simulink model "MMMS_v3"  (R2024b)
settings: Solver=VariableStepAuto  StartTime=0.0  StopTime=60  FixedStep=0.001  RelTol=1e-3
InitFcn:
  | %rho_0t=[0.29;0.29;0.29]; %m
  | %V_0t=[-0.001;-0.001;0];%[-0.0005;-0.0005;0];
  | %w_t=[0;0;-0.002];
  | 
  | 
  | %rho_0t=[0.3;0.3;0.2]; %m
  | %V_0t=[-0.001;-0.001;0];%[-0.0005;-0.0005;0];
  | %w_t=[0;0;-0.001];
values from neighbouring files (symbols this model uses):
  Dt = 0.1    [main_EKF.m]
  Fake_Manip_grad = -0.2.*eye(7)    [Initiate_FQ.m]
  g_cm = zeros(4,4,n)    [Initiate_KUKA_inv.m]    (also in Main_MMMS.m; test_KUKA_elements.m)
  g_It00 = [eye(3) rho_It;0 0 0 1]    [main_EKF.m]
  iota0 = eye(6,6)    [Initiate_KUKA_inv.m]    (also in Main_MMMS.m; test_KUKA_elements.m)
  K_d = 10*[1.3*eye(3) zeros(3);zeros(3) 0.8*eye(3)]    [Initiate_FQ.m]    (also in Initiate_KUKA_inv.m = 5*[0.7*eye(3) zeros(3);zeros(3) 0.5*eye(3)]; MMMS_Initiate_FQ.m; Main_MMMS.m = 5*[0.7*eye(3) zeros(3);zeros(3) 0.5*eye(3)]; test_KUKA_elements.m = 50*[0.7*eye(3) zeros(3);zeros(3) 0.5*eye(3)])
  K_i = 5*[0.1*eye(3) zeros(3);zeros(3) 0.01*eye(3)]    [Initiate_FQ.m]    (also in Initiate_KUKA_inv.m = 5*[0.01*eye(3) zeros(3);zeros(3) 0.001*eye(3)]; MMMS_Initiate_FQ.m; Main_MMMS.m = 5*[0.01*eye(3) zeros(3);zeros(3) 0.001*eye(3)]; test_KUKA_elements.m = 50*[0.01*eye(3) zeros(3);zeros(3) 0.001*eye(3)])
  K_p = 100*[0.1 0 0 0 0 0;0 0.1 0 0 0 0; 0 0 0.1 0 0 0; 0 0 0 0.01 0 0 ... (first row only)    [Initiate_FQ.m]    (also in Initiate_KUKA_inv.m = 5*[0.1 0 0 0 0 0;0 0.1 0 0 0 0; 0 0 0.1 0 0 0; 0 0 0 0.01 0 ; MMMS_Initiate_FQ.m; Main_MMMS.m = 5*[0.1 0 0 0 0 0;0 0.1 0 0 0 0; 0 0 0.1 0 0 0; 0 0 0 0.01 0 ; test_KUKA_elements.m = 50*[0.1 0 0 0 0 0;0 0.1 0 0 0 0; 0 0 0.1 0 0 0; 0 0 0 0.01 0)
  K_w = 200*eye(7)    [Initiate_FQ.m]    (also in MMMS_Initiate_FQ.m)
  K_wd = 2*eye(7)    [Initiate_FQ.m]    (also in MMMS_Initiate_FQ.m)
  m = randn(s,total_time_steps,6)*chol(R)    [main_EKF.m]
  M0 = M_temp.M0.data(:,:,1)    [Initiate_FQ.m]    (also in MMMS_Initiate_FQ.m; test_KUKA_elements.m)
  m0 = robot.Bodies{1,n+1}.Mass    [Initiate_KUKA_inv.m]    (also in Main_MMMS.m; test_KUKA_elements.m)
  m0_frak = diag_M(1:6,1:6)    [Initiate_KUKA_inv.m]    (also in Main_MMMS.m; make_uncertain.m = diag_M_unc(1:6,1:6); test_KUKA_elements.m)
  M0m = M_temp.M0m.data(:,:,1)    [Initiate_FQ.m]    (also in MMMS_Initiate_FQ.m; test_KUKA_elements.m)
  m_diag = diag_M(7:end,7:end)    [Initiate_KUKA_inv.m]    (also in Main_MMMS.m; make_uncertain.m = diag_M_unc(7:end,7:end); test_KUKA_elements.m)
  M_t = (((Adjoint(g_It))'\M_t_body)/(Adjoint(g_It)))    [Initiate_FQ.m]    (also in Initiate_KUKA_inv.m = [eye(3)*mt zeros(3); zeros(3) eye(3)*80]; MMMS_Initiate_FQ.m; Main_MMMS.m = [eye(3)*mt zeros(3); zeros(3) eye(3)*80]; test_KUKA_elements.m = [eye(3)*mt zeros(3); zeros(3) eye(3)*80])
  M_t_body = [eye(3)*mt zeros(3); zeros(3) eye(3)*0.416667]    [Initiate_FQ.m]    (also in MMMS_Initiate_FQ.m)
  mm = zeros(1,n)    [Initiate_KUKA_inv.m]    (also in Main_MMMS.m; test_KUKA_elements.m)
  mu = P0    [Initiate_FQ.m]    (also in Initiate_KUKA_inv.m = zeros(6,1); MMMS_Initiate_FQ.m; Main_MMMS.m = zeros(6,1); make_uncertain.m = P0_unc)
  mu_t = inv((Adjoint(g_It))')*M_t_body*[V_It;w_t]    [Initiate_FQ.m]    (also in Initiate_KUKA_inv.m = M_t*[V_0t;w_t]; MMMS_Initiate_FQ.m; Main_MMMS.m = M_t*[V_0t;w_t]; make_uncertain.m = inv((Adjoint(g_It))')*M_t_body_unc*[V_It;w_t])
  noise_st = 0.000005    (= 5e-06)    [main_EKF.m]
  q_dot_m = [0;0;0;0;0;0;0]    [Initiate_FQ.m]    (also in Initiate_KUKA_inv.m; MMMS_Initiate_FQ.m; Main_MMMS.m; test_KUKA_elements.m = [0])
  q_m = [0.2;1.2;0.3;2.5;0.5;1.5;0.6]    [Initiate_FQ.m]    (also in Initiate_KUKA_inv.m = [0;0;0;0;0;0;0]; MMMS_Initiate_FQ.m = [0.2;0.2;0.3;0.5;0.5;0.5;0.6]; Main_MMMS.m = [0;0;0;0;0;0;0]; test_KUKA_elements.m = [0.2;1.2;0.3;1.8;0.5;1.3;0.6])
  rho_It = [0;0;1.7]    [Initiate_FQ.m]    (also in MMMS_Initiate_FQ.m)
  s = RandStream.create('mrg32k3a','NumStreams',1)    [main_EKF.m]
  sc_size = 1    [Initiate_KUKA_inv.m]    (also in Main_MMMS.m; test_KUKA_elements.m)
  V_It = [0.0005;0.0005;0]    [Initiate_FQ.m]    (also in MMMS_Initiate_FQ.m = [0.001;0.001;0])
  Xi_m_matrix = zeros(6*n,n)    [Initiate_KUKA_inv.m]    (also in Main_MMMS.m)
undefined symbols (not defined in the file or in its folder): g_cm0, I0, Im, Mm, X, Xi_m, Y, Z
libraries: nesl_utility x314, sm_lib x231, robotcorelib x30, simulink x12
(part 7 of 13)

== system MMMS_v3/MMS4/Spacecraft ==
  Base1 : sm_lib/Body Elements/Brick Solid  BrickDimensions=[sc_size,sc_size,sc_size]  BrickDimensionsUnits=m  ExportEntireGeometry=off  InertiaType=Custom  BasedOnType=Mass  Density=1000  DensityUnits=kg/m^3  Mass=0  MassUnits=kg  CenterOfMass=[0 0 0]  CenterOfMassUnits=m  MomentsOfInertia=[0 0 0]  MomentsOfInertiaUnits=kg*m^2  ProductsOfInertia=[0 0 0]  ProductsOfInertiaUnits=kg*m^2  GraphicType=FromGeometry  MarkerShape=Sphere  MarkerSize=10  GraphicVisPropType=SimpleVisualProperties  GraphicDiffuseColor=[0.8 0.8 0.8]  GraphicOpacity=1  GraphicSpecularColor=[0.5 0.5 0.5 1.0]  GraphicAmbientColor=[0.15 0.15 0.15 1.0]  GraphicEmissiveColor=[0.0 0.0 0.0 1.0]  GraphicShininess=75  DoExposeReferenceFrame=on  SerializedFrames=<Frames><Frame><Id>Frame1</Id><Value><Name>F1</Name><Origin><Source>GeometricFeature</Source><FeatureName>+z surface</FeatureName></Origin><PrimaryAxis><DefinedDirection>+X</DefinedDirection><Source>ReferenceFrame</Source><SourceDirection>+X</SourceDirection><FeatureName></FeatureName></PrimaryAxis><SecondaryAxis><DefinedDirection>+Z</DefinedDirection><Source>ReferenceFrame</Source><SourceDirection>+Z</SourceDirection><FeatureName></FeatureName></SecondaryAxis></Value></Frame></Frames>
  Base2 : sm_lib/Body Elements/Brick Solid  Commented=on  BrickDimensions=[sc_size,sc_size,sc_size]  BrickDimensionsUnits=m  ExportEntireGeometry=off  InertiaType=CalculateFromGeometry  BasedOnType=Mass  Density=1000  DensityUnits=kg/m^3  Mass=10  MassUnits=kg  CenterOfMass=[0 0 0]  CenterOfMassUnits=m  MomentsOfInertia=[0 0 0]  MomentsOfInertiaUnits=kg*m^2  ProductsOfInertia=[0 0 0]  ProductsOfInertiaUnits=kg*m^2  GraphicType=FromGeometry  MarkerShape=Sphere  MarkerSize=10  GraphicVisPropType=SimpleVisualProperties  GraphicDiffuseColor=[0.5 0.5 0.5]  GraphicOpacity=1.0  GraphicSpecularColor=[0.5 0.5 0.5 1.0]  GraphicAmbientColor=[0.15 0.15 0.15 1.0]  GraphicEmissiveColor=[0.0 0.0 0.0 1.0]  GraphicShininess=75  DoExposeReferenceFrame=on  SerializedFrames=<Frames><Frame><Id>Frame1</Id><Value><Name>F1</Name><Origin><Source>GeometricFeature</Source><FeatureName>+z surface</FeatureName></Origin><PrimaryAxis><DefinedDirection>+X</DefinedDirection><Source>ReferenceFrame</Source><SourceDirection>+X</SourceDirection><FeatureName></FeatureName></PrimaryAxis><SecondaryAxis><DefinedDirection>+Z</DefinedDirection><Source>ReferenceFrame</Source><SourceDirection>+Z</SourceDirection><FeatureName></FeatureName></SecondaryAxis></Value></Frame></Frames>
  Cylindrical Solid : sm_lib/Body Elements/Cylindrical Solid  CylinderRadius=0.09  CylinderRadiusUnits=m  CylinderLength=0.15  CylinderLengthUnits=m  ExportEntireGeometry=off  InertiaType=CalculateFromGeometry  BasedOnType=Density  Density=0  DensityUnits=kg/m^3  Mass=1  MassUnits=kg  CenterOfMass=[0 0 0]  CenterOfMassUnits=m  MomentsOfInertia=[1 1 1]  MomentsOfInertiaUnits=kg*m^2  ProductsOfInertia=[0 0 0]  ProductsOfInertiaUnits=kg*m^2  GraphicType=FromGeometry  MarkerShape=Sphere  MarkerSize=10  GraphicVisPropType=SimpleVisualProperties  GraphicDiffuseColor=[0.8 0.8 0.8]  GraphicOpacity=1.0  GraphicSpecularColor=[0.5 0.5 0.5 1.0]  GraphicAmbientColor=[0.15 0.15 0.15 1.0]  GraphicEmissiveColor=[0.0 0.0 0.0 1.0]  GraphicShininess=75  DoExposeReferenceFrame=on  SerializedFrames=<Frames><Frame><Id>Frame1</Id><Value><Name>F1</Name><Origin><Source>GeometricFeature</Source><FeatureName>top surface</FeatureName></Origin><PrimaryAxis><DefinedDirection>+Z</DefinedDirection><Source>ReferenceFrame</Source><SourceDirection>+Z</SourceDirection><FeatureName></FeatureName></PrimaryAxis><SecondaryAxis><DefinedDirection>+X</DefinedDirection><Source>ReferenceFrame</Source><SourceDirection>+X</SourceDirection><FeatureName></FeatureName></SecondaryAxis></Value></Frame></Frames>
  Inertia : sm_lib/Body Elements/Inertia  InertiaType=Custom  Mass=mm(7)  MassUnits=kg  CenterOfMass=[0, 0, 0]  CenterOfMassUnits=m  MomentsOfInertia=[Im(1,1,7) Im(2,2,7) Im(3,3,7)]  MomentsOfInertiaUnits=kg*m^2  ProductsOfInertia=[Im(3,2,7) Im(3,1,7) Im(2,1,7)]  ProductsOfInertiaUnits=kg*m^2  GraphicType=None  MarkerShape=Inertia  MarkerSize=20  GraphicVisPropType=SimpleVisualProperties  GraphicDiffuseColor=[0.5 0.5 0.5]  GraphicOpacity=1.0  GraphicSpecularColor=[0.5 0.5 0.5 1.0]  GraphicAmbientColor=[0.15 0.15 0.15 1.0]  GraphicEmissiveColor=[0.0 0.0 0.0 1.0]  GraphicShininess=75
  Planar Joint : sm_lib/Joints/Planar Joint  JointMode=Normal  CompositeWrenchDir=FollowerOnBase  CompositeWrenchFrame=BaseFrame  SenseConstraintForce=off  SenseConstraintTorque=off  SenseTotalForce=off  SenseTotalTorque=off  PxPositionTargetSpecify=on  PxPositionTargetPriority=High  PxPositionTargetValue=0.75  PxPositionTargetValueUnits=m  PxVelocityTargetSpecify=off  PxVelocityTargetPriority=High  PxVelocityTargetValue=0  PxVelocityTargetValueUnits=m/s  PxEquilibriumPosition=0  PxEquilibriumPositionUnits=m  PxSpringStiffness=0  PxSpringStiffnessUnits=N/m  PxDampingCoefficient=0  PxDampingCoefficientUnits=N/(m/s)  PxLowerLimitSpecify=off  PxLowerLimitBound=-1  PxLowerLimitBoundUnits=m  PxLowerLimitStiffness=1e6  PxLowerLimitStiffnessUnits=N/m  PxLowerLimitDamping=1e3  PxLowerLimitDampingUnits=N/(m/s)  PxLowerLimitTransitionRegionWidth=1e-4  PxLowerLimitTransitionRegionWidthUnits=m  PxUpperLimitSpecify=off  PxUpperLimitBound=1  PxUpperLimitBoundUnits=m  PxUpperLimitStiffness=1e6  PxUpperLimitStiffnessUnits=N/m  PxUpperLimitDamping=1e3  PxUpperLimitDampingUnits=N/(m/s)  PxUpperLimitTransitionRegionWidth=1e-4  PxUpperLimitTransitionRegionWidthUnits=m  PxTorqueActuationMode=NoTorque  PxMotionActuationMode=ComputedMotion  PxSensePosition=off  PxSenseVelocity=off  PxSenseAcceleration=off  PxSenseTorqueForce=off  PxSenseLowerLimitTorqueForce=off  PxSenseUpperLimitTorqueForce=off  PyPositionTargetSpecify=on  PyPositionTargetPriority=High  PyPositionTargetValue=0  PyPositionTargetValueUnits=m  PyVelocityTargetSpecify=off  PyVelocityTargetPriority=High  PyVelocityTargetValue=0  PyVelocityTargetValueUnits=m/s  PyEquilibriumPosition=0  PyEquilibriumPositionUnits=m  PySpringStiffness=0  PySpringStiffnessUnits=N/m  PyDampingCoefficient=0  PyDampingCoefficientUnits=N/(m/s)  PyLowerLimitSpecify=off  PyLowerLimitBound=-1  PyLowerLimitBoundUnits=m  PyLowerLimitStiffness=1e6  PyLowerLimitStiffnessUnits=N/m  PyLowerLimitDamping=1e3  PyLowerLimitDampingUnits=N/(m/s)  PyLowerLimitTransitionRegionWidth=1e-4  PyLowerLimitTransitionRegionWidthUnits=m  PyUpperLimitSpecify=off  PyUpperLimitBound=1  PyUpperLimitBoundUnits=m  PyUpperLimitStiffness=1e6  PyUpperLimitStiffnessUnits=N/m  PyUpperLimitDamping=1e3  PyUpperLimitDampingUnits=N/(m/s)  PyUpperLimitTransitionRegionWidth=1e-4  PyUpperLimitTransitionRegionWidthUnits=m  PyTorqueActuationMode=NoTorque  PyMotionActuationMode=ComputedMotion  PySensePosition=off  PySenseVelocity=off  PySenseAcceleration=off  PySenseTorqueForce=off  PySenseLowerLimitTorqueForce=off  PySenseUpperLimitTorqueForce=off  RzPositionTargetSpecify=off  RzPositionTargetPriority=High  RzPositionTargetValue=-1  RzPositionTargetValueUnits=deg  RzVelocityTargetSpecify=off  RzVelocityTargetPriority=High  RzVelocityTargetValue=0  RzVelocityTargetValueUnits=deg/s  RzEquilibriumPosition=0  RzEquilibriumPositionUnits=deg  RzSpringStiffness=0  RzSpringStiffnessUnits=N*m/deg  RzDampingCoefficient=0  RzDampingCoefficientUnits=N*m/(deg/s)  RzLowerLimitSpecify=off  RzLowerLimitBound=-90  RzLowerLimitBoundUnits=deg  RzLowerLimitStiffness=1e4  RzLowerLimitStiffnessUnits=N*m/deg  RzLowerLimitDamping=10  RzLowerLimitDampingUnits=N*m/(deg/s)  RzLowerLimitTransitionRegionWidth=0.1  RzLowerLimitTransitionRegionWidthUnits=deg  RzUpperLimitSpecify=off  RzUpperLimitBound=90  RzUpperLimitBoundUnits=deg  RzUpperLimitStiffness=1e4  RzUpperLimitStiffnessUnits=N*m/deg  RzUpperLimitDamping=10  RzUpperLimitDampingUnits=N*m/(deg/s)  RzUpperLimitTransitionRegionWidth=0.1  RzUpperLimitTransitionRegionWidthUnits=deg  RzTorqueActuationMode=NoTorque  RzMotionActuationMode=ComputedMotion  RzSensePosition=off  RzSenseVelocity=off  RzSenseAcceleration=off  RzSenseTorqueForce=off  RzSenseLowerLimitTorqueForce=off  RzSenseUpperLimitTorqueForce=off
  Visual : sm_lib/Body Elements/File Solid  Commented=on  ExtGeomFileName=iiwa_description/meshes/iiwa7/visual/link_1.stl  UnitType=Custom  ExtGeomFileUnits=m  StepReaderType=HEX  ExportConvexHullGeometry=off  InertiaType=Custom  BasedOnType=DensityFromFile  Density=1000  DensityUnits=kg/m^3  Mass=0  MassUnits=kg  CenterOfMass=[0, 0, 0]  CenterOfMassUnits=m  MomentsOfInertia=[0, 0, 0]  MomentsOfInertiaUnits=kg*m^2  ProductsOfInertia=[0, 0, 0]  ProductsOfInertiaUnits=kg*m^2  GraphicType=FromGeometry  MarkerShape=Sphere  MarkerSize=10  GraphicVisPropType=SimpleVisualProperties  GraphicDiffuseColor=[1, 0.423529411765, 0.0392156862745]  GraphicOpacity=1  GraphicSpecularColor=[0.5 0.5 0.5 1.0]  GraphicAmbientColor=[0.15 0.15 0.15 1.0]  GraphicEmissiveColor=[0.0 0.0 0.0 1.0]  GraphicShininess=75  DoExposeReferenceFrame=on  SerializedFrames=<Frames/>
  VisualOriginTransform : sm_lib/Frames and Transforms/Rigid Transform  RotationMethod=RotationSequence  FollAlignAxisA=+X  BaseAlignAxisA=+Y  FollAlignAxisB=+Y  BaseAlignAxisB=+Z  RotationStandardAxis=+Z  RotationAngle=0.0  RotationAngleUnits=deg  RotationArbitraryAxis=[0 0 1]  RotationSequenceAxes=BaseAxes  RotationSequence=XYZ  RotationSequenceAngles=[0, 0, 0]  RotationSequenceAnglesUnits=rad  RotationMatrix=[1 0 0; 0 1 0; 0 0 1]  Quaternion=[1 0 0 0]  TranslationMethod=Cartesian  TranslationCartesianOffset=[0, 0, -0.15]  TranslationCartesianOffsetUnits=m  TranslationStandardAxis=+Z  TranslationStandardOffset=0  TranslationStandardOffsetUnits=m  TranslationROffset=0  TranslationROffsetUnits=m  TranslationThetaOffset=0  TranslationThetaOffsetUnits=deg  TranslationZOffset=0  TranslationZOffsetUnits=m
  iiwa_joint_2_OriginTransform : sm_lib/Frames and Transforms/Rigid Transform  RotationMethod=RotationMatrix  FollAlignAxisA=+X  BaseAlignAxisA=+Y  FollAlignAxisB=+Y  BaseAlignAxisB=+Z  RotationStandardAxis=+Z  RotationAngle=0.0  RotationAngleUnits=deg  RotationArbitraryAxis=[0 0 1]  RotationSequenceAxes=BaseAxes  RotationSequence=XYZ  RotationSequenceAngles=[1.57079632679, 0, 3.14159265359]  RotationSequenceAnglesUnits=rad  RotationMatrix=g_cm(1:3,1:3,7)  Quaternion=[1 0 0 0]  TranslationMethod=Cartesian  TranslationCartesianOffset=g_cm(1:3,4,7)'  TranslationCartesianOffsetUnits=m  TranslationStandardAxis=+Z  TranslationStandardOffset=0  TranslationStandardOffsetUnits=m  TranslationROffset=0  TranslationROffsetUnits=m  TranslationThetaOffset=0  TranslationThetaOffsetUnits=deg  TranslationZOffset=0  TranslationZOffsetUnits=m
  iiwa_joint_2_OriginTransform1 : sm_lib/Frames and Transforms/Rigid Transform  RotationMethod=RotationMatrix  FollAlignAxisA=+X  BaseAlignAxisA=+Y  FollAlignAxisB=+Y  BaseAlignAxisB=+Z  RotationStandardAxis=+Z  RotationAngle=0.0  RotationAngleUnits=deg  RotationArbitraryAxis=[0 0 1]  RotationSequenceAxes=BaseAxes  RotationSequence=XYZ  RotationSequenceAngles=[1.57079632679, 0, 3.14159265359]  RotationSequenceAnglesUnits=rad  RotationMatrix=g_cm(1:3,1:3,7)  Quaternion=[1 0 0 0]  TranslationMethod=Cartesian  TranslationCartesianOffset=g_cm(1:3,4,7)'  TranslationCartesianOffsetUnits=m  TranslationStandardAxis=+Z  TranslationStandardOffset=0  TranslationStandardOffsetUnits=m  TranslationROffset=0  TranslationROffsetUnits=m  TranslationThetaOffset=0  TranslationThetaOffsetUnits=deg  TranslationZOffset=0  TranslationZOffsetUnits=m
  F : PMIOPort  Side=Left
  F1 : PMIOPort  Port=2  Side=Right
  F3 : PMIOPort  Port=3  Side=Left
  connections:
  F3/RConn1 -- Planar Joint/LConn1
  iiwa_joint_2_OriginTransform/LConn1 -- Cylindrical Solid/LConn1 -- F1/RConn1
  iiwa_joint_2_OriginTransform1/LConn1 -- Inertia/RConn1 -- iiwa_joint_2_OriginTransform/RConn1 -- VisualOriginTransform/LConn1 -- F/RConn1
  Base1/RConn1 -- VisualOriginTransform/RConn1
  Planar Joint/RConn1 -- iiwa_joint_2_OriginTransform1/RConn1

== system MMMS_v3/MMS4/join//link 1 ==
  iiwa_joint_1 : sm_lib/Joints/Revolute Joint  JointMode=Normal  CompositeWrenchDir=FollowerOnBase  CompositeWrenchFrame=BaseFrame  SenseConstraintForce=off  SenseConstraintTorque=off  SenseTotalForce=off  SenseTotalTorque=off  PositionTargetSpecify=on  PositionTargetPriority=High  PositionTargetValue=q_m(7)  PositionTargetValueUnits=rad  VelocityTargetSpecify=on  VelocityTargetPriority=High  VelocityTargetValue=q_dot_m(7)  VelocityTargetValueUnits=rad/s  EquilibriumPosition=0  EquilibriumPositionUnits=deg  SpringStiffness=0  SpringStiffnessUnits=N*m/deg  DampingCoefficient=0  DampingCoefficientUnits=kg*m^2/(rad*s)  LowerLimitSpecify=off  LowerLimitBound=-2.96705972839  LowerLimitBoundUnits=rad  LowerLimitStiffness=1e4  LowerLimitStiffnessUnits=N*m/deg  LowerLimitDamping=10  LowerLimitDampingUnits=N*m/(deg/s)  LowerLimitTransitionRegionWidth=0.1  LowerLimitTransitionRegionWidthUnits=deg  UpperLimitSpecify=off  UpperLimitBound=2.96705972839  UpperLimitBoundUnits=rad  UpperLimitStiffness=1e4  UpperLimitStiffnessUnits=N*m/deg  UpperLimitDamping=10  UpperLimitDampingUnits=N*m/(deg/s)  UpperLimitTransitionRegionWidth=0.1  UpperLimitTransitionRegionWidthUnits=deg  TorqueActuationMode=InputTorque  MotionActuationMode=ComputedMotion  SensePosition=on  SenseVelocity=on  SenseAcceleration=on  SenseTorqueForce=off  SenseLowerLimitTorqueForce=off  SenseUpperLimitTorqueForce=off
  iiwa_link_1 : Subsystem
  b : PMIOPort  Side=Left
  f1 : PMIOPort  Port=2  Side=Left
  F1 : PMIOPort  Port=3  Side=Right
  q1 : PMIOPort  Port=4  Side=Right
  qd1 : PMIOPort  Port=5  Side=Right
  qdd1 : PMIOPort  Port=6  Side=Right
  connections:
  F1/RConn1 -- iiwa_link_1/RConn1
  iiwa_joint_1/RConn4 -- qdd1/RConn1
  iiwa_joint_1/RConn3 -- qd1/RConn1
  f1/RConn1 -- iiwa_joint_1/LConn2
  iiwa_joint_1/RConn2 -- q1/RConn1
  iiwa_joint_1/RConn1 -- b/RConn1
  iiwa_link_1/LConn1 -- iiwa_joint_1/LConn1

== system MMMS_v3/MMS4/joint//link2 ==
  iiwa_joint_2 : sm_lib/Joints/Revolute Joint  JointMode=Normal  CompositeWrenchDir=FollowerOnBase  CompositeWrenchFrame=BaseFrame  SenseConstraintForce=off  SenseConstraintTorque=off  SenseTotalForce=off  SenseTotalTorque=off  PositionTargetSpecify=on  PositionTargetPriority=High  PositionTargetValue=q_m(6)  PositionTargetValueUnits=rad  VelocityTargetSpecify=on  VelocityTargetPriority=High  VelocityTargetValue=q_dot_m(6)  VelocityTargetValueUnits=rad/s  EquilibriumPosition=0  EquilibriumPositionUnits=deg  SpringStiffness=0  SpringStiffnessUnits=N*m/deg  DampingCoefficient=0  DampingCoefficientUnits=kg*m^2/(rad*s)  LowerLimitSpecify=off  LowerLimitBound=-2.09439510239  LowerLimitBoundUnits=rad  LowerLimitStiffness=1e4  LowerLimitStiffnessUnits=N*m/deg  LowerLimitDamping=10  LowerLimitDampingUnits=N*m/(deg/s)  LowerLimitTransitionRegionWidth=0.1  LowerLimitTransitionRegionWidthUnits=deg  UpperLimitSpecify=off  UpperLimitBound=2.09439510239  UpperLimitBoundUnits=rad  UpperLimitStiffness=1e4  UpperLimitStiffnessUnits=N*m/deg  UpperLimitDamping=10  UpperLimitDampingUnits=N*m/(deg/s)  UpperLimitTransitionRegionWidth=0.1  UpperLimitTransitionRegionWidthUnits=deg  TorqueActuationMode=InputTorque  MotionActuationMode=ComputedMotion  SensePosition=on  SenseVelocity=on  SenseAcceleration=on  SenseTorqueForce=off  SenseLowerLimitTorqueForce=off  SenseUpperLimitTorqueForce=off
  iiwa_link_2 : Subsystem
  b : PMIOPort  Side=Left
  F1 : PMIOPort  Port=2  Side=Right
  f2 : PMIOPort  Port=3  Side=Left
  q2 : PMIOPort  Port=4  Side=Right
  qd2 : PMIOPort  Port=5  Side=Right
  qdd2 : PMIOPort  Port=6  Side=Right
  connections:
  iiwa_joint_2/RConn2 -- q2/RConn1
  f2/RConn1 -- iiwa_joint_2/LConn2
  iiwa_joint_2/RConn1 -- b/RConn1
  iiwa_joint_2/RConn4 -- qdd2/RConn1
  F1/RConn1 -- iiwa_link_2/RConn1
  iiwa_link_2/LConn1 -- iiwa_joint_2/LConn1
  iiwa_joint_2/RConn3 -- qd2/RConn1

== system MMMS_v3/MMS4/joint//link3 ==
  iiwa_joint_3 : sm_lib/Joints/Revolute Joint  JointMode=Normal  CompositeWrenchDir=FollowerOnBase  CompositeWrenchFrame=BaseFrame  SenseConstraintForce=off  SenseConstraintTorque=off  SenseTotalForce=off  SenseTotalTorque=off  PositionTargetSpecify=on  PositionTargetPriority=High  PositionTargetValue=q_m(5)  PositionTargetValueUnits=rad  VelocityTargetSpecify=on  VelocityTargetPriority=High  VelocityTargetValue=q_dot_m(5)  VelocityTargetValueUnits=rad/s  EquilibriumPosition=0  EquilibriumPositionUnits=deg  SpringStiffness=0  SpringStiffnessUnits=N*m/deg  DampingCoefficient=0  DampingCoefficientUnits=kg*m^2/(rad*s)  LowerLimitSpecify=off  LowerLimitBound=-2.96705972839  LowerLimitBoundUnits=rad  LowerLimitStiffness=1e4  LowerLimitStiffnessUnits=N*m/deg  LowerLimitDamping=10  LowerLimitDampingUnits=N*m/(deg/s)  LowerLimitTransitionRegionWidth=0.1  LowerLimitTransitionRegionWidthUnits=deg  UpperLimitSpecify=off  UpperLimitBound=2.96705972839  UpperLimitBoundUnits=rad  UpperLimitStiffness=1e4  UpperLimitStiffnessUnits=N*m/deg  UpperLimitDamping=10  UpperLimitDampingUnits=N*m/(deg/s)  UpperLimitTransitionRegionWidth=0.1  UpperLimitTransitionRegionWidthUnits=deg  TorqueActuationMode=InputTorque  MotionActuationMode=ComputedMotion  SensePosition=on  SenseVelocity=on  SenseAcceleration=on  SenseTorqueForce=off  SenseLowerLimitTorqueForce=off  SenseUpperLimitTorqueForce=off
  iiwa_link_3 : Subsystem
  b : PMIOPort  Side=Left
  F1 : PMIOPort  Port=2  Side=Right
  f3 : PMIOPort  Port=3  Side=Left
  q3 : PMIOPort  Port=4  Side=Right
  qd3 : PMIOPort  Port=5  Side=Right
  qdd3 : PMIOPort  Port=6  Side=Right
  connections:
  iiwa_joint_3/RConn1 -- b/RConn1
  f3/RConn1 -- iiwa_joint_3/LConn2
  F1/RConn1 -- iiwa_link_3/RConn1
  iiwa_joint_3/RConn2 -- q3/RConn1
  iiwa_joint_3/RConn3 -- qd3/RConn1
  iiwa_joint_3/RConn4 -- qdd3/RConn1
  iiwa_link_3/LConn1 -- iiwa_joint_3/LConn1

== system MMMS_v3/MMS4/joint//link4 ==
  iiwa_joint_4 : sm_lib/Joints/Revolute Joint  JointMode=Normal  CompositeWrenchDir=FollowerOnBase  CompositeWrenchFrame=BaseFrame  SenseConstraintForce=off  SenseConstraintTorque=off  SenseTotalForce=off  SenseTotalTorque=off  PositionTargetSpecify=on  PositionTargetPriority=High  PositionTargetValue=q_m(4)  PositionTargetValueUnits=rad  VelocityTargetSpecify=on  VelocityTargetPriority=High  VelocityTargetValue=q_dot_m(4)  VelocityTargetValueUnits=rad/s  EquilibriumPosition=0  EquilibriumPositionUnits=deg  SpringStiffness=0  SpringStiffnessUnits=N*m/deg  DampingCoefficient=0  DampingCoefficientUnits=kg*m^2/(rad*s)  LowerLimitSpecify=off  LowerLimitBound=-2.09439510239  LowerLimitBoundUnits=rad  LowerLimitStiffness=1e4  LowerLimitStiffnessUnits=N*m/deg  LowerLimitDamping=10  LowerLimitDampingUnits=N*m/(deg/s)  LowerLimitTransitionRegionWidth=0.1  LowerLimitTransitionRegionWidthUnits=deg  UpperLimitSpecify=off  UpperLimitBound=2.09439510239  UpperLimitBoundUnits=rad  UpperLimitStiffness=1e4  UpperLimitStiffnessUnits=N*m/deg  UpperLimitDamping=10  UpperLimitDampingUnits=N*m/(deg/s)  UpperLimitTransitionRegionWidth=0.1  UpperLimitTransitionRegionWidthUnits=deg  TorqueActuationMode=InputTorque  MotionActuationMode=ComputedMotion  SensePosition=on  SenseVelocity=on  SenseAcceleration=on  SenseTorqueForce=off  SenseLowerLimitTorqueForce=off  SenseUpperLimitTorqueForce=off
  iiwa_link_4 : Subsystem
  b : PMIOPort  Side=Left
  F1 : PMIOPort  Port=2  Side=Right
  f4 : PMIOPort  Port=3  Side=Left
  q4 : PMIOPort  Port=4  Side=Right
  qd4 : PMIOPort  Port=5  Side=Right
  qdd4 : PMIOPort  Port=6  Side=Right
  connections:
  iiwa_joint_4/RConn4 -- qdd4/RConn1
  iiwa_joint_4/RConn1 -- b/RConn1
  iiwa_joint_4/RConn2 -- q4/RConn1
  F1/RConn1 -- iiwa_link_4/RConn1
  f4/RConn1 -- iiwa_joint_4/LConn2
  iiwa_joint_4/RConn3 -- qd4/RConn1
  iiwa_link_4/LConn1 -- iiwa_joint_4/LConn1

== system MMMS_v3/MMS4/joint//link5 ==
  iiwa_joint_5 : sm_lib/Joints/Revolute Joint  JointMode=Normal  CompositeWrenchDir=FollowerOnBase  CompositeWrenchFrame=BaseFrame  SenseConstraintForce=off  SenseConstraintTorque=off  SenseTotalForce=off  SenseTotalTorque=off  PositionTargetSpecify=on  PositionTargetPriority=High  PositionTargetValue=q_m(3)  PositionTargetValueUnits=rad  VelocityTargetSpecify=on  VelocityTargetPriority=High  VelocityTargetValue=q_dot_m(3)  VelocityTargetValueUnits=rad/s  EquilibriumPosition=0  EquilibriumPositionUnits=rad  SpringStiffness=0  SpringStiffnessUnits=N*m/rad  DampingCoefficient=0  DampingCoefficientUnits=kg*m^2/(rad*s)  LowerLimitSpecify=off  LowerLimitBound=-2.96705972839  LowerLimitBoundUnits=rad  LowerLimitStiffness=1e4  LowerLimitStiffnessUnits=N*m/deg  LowerLimitDamping=10  LowerLimitDampingUnits=N*m/(deg/s)  LowerLimitTransitionRegionWidth=0.1  LowerLimitTransitionRegionWidthUnits=deg  UpperLimitSpecify=off  UpperLimitBound=2.96705972839  UpperLimitBoundUnits=rad  UpperLimitStiffness=1e4  UpperLimitStiffnessUnits=N*m/deg  UpperLimitDamping=10  UpperLimitDampingUnits=N*m/(deg/s)  UpperLimitTransitionRegionWidth=0.1  UpperLimitTransitionRegionWidthUnits=deg  TorqueActuationMode=InputTorque  MotionActuationMode=ComputedMotion  SensePosition=on  SenseVelocity=on  SenseAcceleration=on  SenseTorqueForce=off  SenseLowerLimitTorqueForce=off  SenseUpperLimitTorqueForce=off
  iiwa_link_5 : Subsystem
  b : PMIOPort  Side=Left
  F1 : PMIOPort  Port=2  Side=Right
  f5 : PMIOPort  Port=3  Side=Left
  q5 : PMIOPort  Port=4  Side=Right
  qd5 : PMIOPort  Port=5  Side=Right
  qdd5 : PMIOPort  Port=6  Side=Right
  connections:
  F1/RConn1 -- iiwa_link_5/RConn1
  f5/RConn1 -- iiwa_joint_5/LConn2
  iiwa_joint_5/RConn3 -- qd5/RConn1
  iiwa_link_5/LConn1 -- iiwa_joint_5/LConn1
  iiwa_joint_5/RConn4 -- qdd5/RConn1
  iiwa_joint_5/RConn2 -- q5/RConn1
  iiwa_joint_5/RConn1 -- b/RConn1

== system MMMS_v3/MMS4/joint//link6 ==
  PS-Simulink Converter1 : nesl_utility/PS-Simulink Converter  PhysicalDomain=network_engine_domain  SubClassName=ps_output  LeftPortType=input  RightPortType=output  PseudoPeriodic=off  Frequencies=[]  VectorFormat=1-D array  Unit=inherit  AffineConversion=off
  Scope : Scope
  iiwa_joint_6 : sm_lib/Joints/Revolute Joint  JointMode=Normal  CompositeWrenchDir=FollowerOnBase  CompositeWrenchFrame=BaseFrame  SenseConstraintForce=off  SenseConstraintTorque=off  SenseTotalForce=off  SenseTotalTorque=off  PositionTargetSpecify=on  PositionTargetPriority=High  PositionTargetValue=q_m(2)  PositionTargetValueUnits=rad  VelocityTargetSpecify=on  VelocityTargetPriority=High  VelocityTargetValue=q_dot_m(2)  VelocityTargetValueUnits=rad/s  EquilibriumPosition=0  EquilibriumPositionUnits=rad  SpringStiffness=0  SpringStiffnessUnits=N*m/rad  DampingCoefficient=0  DampingCoefficientUnits=kg*m^2/(rad*s)  LowerLimitSpecify=off  LowerLimitBound=-2.09439510239  LowerLimitBoundUnits=rad  LowerLimitStiffness=1e4  LowerLimitStiffnessUnits=N*m/deg  LowerLimitDamping=10  LowerLimitDampingUnits=N*m/(deg/s)  LowerLimitTransitionRegionWidth=0.1  LowerLimitTransitionRegionWidthUnits=deg  UpperLimitSpecify=off  UpperLimitBound=2.09439510239  UpperLimitBoundUnits=rad  UpperLimitStiffness=1e4  UpperLimitStiffnessUnits=N*m/deg  UpperLimitDamping=10  UpperLimitDampingUnits=N*m/(deg/s)  UpperLimitTransitionRegionWidth=0.1  UpperLimitTransitionRegionWidthUnits=deg  TorqueActuationMode=InputTorque  MotionActuationMode=ComputedMotion  SensePosition=on  SenseVelocity=on  SenseAcceleration=on  SenseTorqueForce=on  SenseLowerLimitTorqueForce=off  SenseUpperLimitTorqueForce=off
  iiwa_link_6 : Subsystem
  b : PMIOPort  Side=Left
  f6 : PMIOPort  Port=2  Side=Left
  F1 : PMIOPort  Port=3  Side=Right
  q6 : PMIOPort  Port=4  Side=Right
  qd6 : PMIOPort  Port=5  Side=Right
  qdd6 : PMIOPort  Port=6  Side=Right
  wires:
  PS-Simulink Converter1/1 -> Scope/1  "q_dot_1 to 3"
  connections:
  iiwa_joint_6/RConn5 -- PS-Simulink Converter1/LConn1
  iiwa_joint_6/RConn2 -- q6/RConn1
  iiwa_joint_6/RConn3 -- qd6/RConn1
  iiwa_joint_6/RConn4 -- qdd6/RConn1
  f6/RConn1 -- iiwa_joint_6/LConn2
  F1/RConn1 -- iiwa_link_6/RConn1
  iiwa_joint_6/RConn1 -- b/RConn1
  iiwa_link_6/LConn1 -- iiwa_joint_6/LConn1

== system MMMS_v3/MMS4/joint//link7 ==
  PS-Simulink Converter1 : nesl_utility/PS-Simulink Converter  PhysicalDomain=network_engine_domain  SubClassName=ps_output  LeftPortType=input  RightPortType=output  PseudoPeriodic=off  Frequencies=[]  VectorFormat=1-D array  Unit=inherit  AffineConversion=off
  Scope : Scope
  iiwa_joint_7 : sm_lib/Joints/Revolute Joint  JointMode=Normal  CompositeWrenchDir=FollowerOnBase  CompositeWrenchFrame=BaseFrame  SenseConstraintForce=off  SenseConstraintTorque=off  SenseTotalForce=off  SenseTotalTorque=off  PositionTargetSpecify=on  PositionTargetPriority=High  PositionTargetValue=q_m(1)  PositionTargetValueUnits=rad  VelocityTargetSpecify=on  VelocityTargetPriority=High  VelocityTargetValue=q_dot_m(1)  VelocityTargetValueUnits=rad/s  EquilibriumPosition=0  EquilibriumPositionUnits=rad  SpringStiffness=0  SpringStiffnessUnits=N*m/rad  DampingCoefficient=0  DampingCoefficientUnits=kg*m^2/(rad*s)  LowerLimitSpecify=off  LowerLimitBound=-3.05432619099  LowerLimitBoundUnits=rad  LowerLimitStiffness=1e4  LowerLimitStiffnessUnits=N*m/deg  LowerLimitDamping=10  LowerLimitDampingUnits=N*m/(deg/s)  LowerLimitTransitionRegionWidth=0.1  LowerLimitTransitionRegionWidthUnits=deg  UpperLimitSpecify=off  UpperLimitBound=3.05432619099  UpperLimitBoundUnits=rad  UpperLimitStiffness=1e4  UpperLimitStiffnessUnits=N*m/deg  UpperLimitDamping=10  UpperLimitDampingUnits=N*m/(deg/s)  UpperLimitTransitionRegionWidth=0.1  UpperLimitTransitionRegionWidthUnits=deg  TorqueActuationMode=InputTorque  MotionActuationMode=ComputedMotion  SensePosition=on  SenseVelocity=on  SenseAcceleration=on  SenseTorqueForce=on  SenseLowerLimitTorqueForce=off  SenseUpperLimitTorqueForce=off
  iiwa_link_7 : Subsystem
  b : PMIOPort  Side=Left
  f7 : PMIOPort  Port=2  Side=Left
  F1 : PMIOPort  Port=3  Side=Right
  q7 : PMIOPort  Port=4  Side=Right
  qd7 : PMIOPort  Port=5  Side=Right
  qdd7 : PMIOPort  Port=6  Side=Right
  wires:
  PS-Simulink Converter1/1 -> Scope/1  "q_dot_1 to 3"
  connections:
  iiwa_joint_7/RConn5 -- PS-Simulink Converter1/LConn1
  iiwa_joint_7/RConn1 -- b/RConn1
  F1/RConn1 -- iiwa_link_7/RConn1
  f7/RConn1 -- iiwa_joint_7/LConn2
  iiwa_joint_7/RConn3 -- qd7/RConn1
  iiwa_joint_7/RConn2 -- q7/RConn1
  iiwa_joint_7/RConn4 -- qdd7/RConn1
  iiwa_link_7/LConn1 -- iiwa_joint_7/LConn1

== system MMMS_v3/Controller23/Filter/Triggered Subsystem ==
  X_pos : Inport
  P_pos : Inport  Port=2
  Z : Inport  Port=3
  Trigger : TriggerPort  VariantControl=(inherit)  ShowOutputPort=on  SampleTimeType=periodic  SampleTime=0.5  InitialTriggerSignalState=positive
  Constant10 : Constant  Value=Dt
  Constant11 : Constant  Value=mu_t
  Constant12 : Constant  Value=noise_st.*eye(6)
  Constant13 : Constant  Value=noise_st.*eye(6)
  MATLAB Function : MATLAB Function  TreatAsAtomicUnit=on
  Mass : Constant  Value=[M_t(4:6,4:6) zeros(3); zeros(3) M_t(1:3,1:3)]
  Scope17 : Scope
  X_pos_out : Outport
  P_pos_out : Outport  Port=2
  wires:
  MATLAB Function/1(X_pos_out) -> X_pos_out/1
  Constant10/1 -> MATLAB Function/2(Dt)
  Mass/1 -> MATLAB Function/3(Mass_matrix)
  Constant13/1 -> MATLAB Function/8(R)
  Constant11/1 -> MATLAB Function/5(mu_vector)
  Constant12/1 -> MATLAB Function/7(Q)
  X_pos/1 -> MATLAB Function/4(X_pos)
  MATLAB Function/2(P_pos_out) -> P_pos_out/1
  P_pos/1 -> MATLAB Function/6(P_pos)
  Z/1 -> MATLAB Function/1(Z)
  Trigger/1 -> Scope17/1

== system MMMS_v3/Feedback Transformation/Inverse Dynamics1/C_hat ==
  note: C_hat
  q_m1 : Inport
  q_dot_m1 : Inport  Port=2
  A : Inport  Port=3
  <Lm0> : Inport  Port=4
  <Lm> : Inport  Port=5
  <M0> : Inport  Port=6
  <M0m> : Inport  Port=7
  <M0>1 : InportShadow  Port=6
  AMA_partial : MATLAB Function  TreatAsAtomicUnit=on
  A_partial : MATLAB Function  TreatAsAtomicUnit=on
  C_hat1 : MATLAB Function  TreatAsAtomicUnit=on
  Constant : Constant  Value=Xi_m
  Lm_partials : Subsystem
  M_partials : Subsystem
  Mm_hat_partial : MATLAB Function  TreatAsAtomicUnit=on
  M0_partial : Outport
  A_partial1 : Outport  Port=2
  C_hat : Outport  Port=3
  tag scope: A_partial=global, M0_partial=global
  wires:
  M_partials/3(Mm_partial) -> Mm_hat_partial/3(Mm_partial)
  Lm_partials/2(Lm0_partial) -> M_partials/3(Lm0_partial)
  q_m1/1 -> Lm_partials/1(q_m), Mm_hat_partial/1(q_m), C_hat1/1(q_m), AMA_partial/1(q_m), A_partial/1(q_m), M_partials/1(q_m)
  <M0m>/1 -> A_partial/5(M0m)
  Lm_partials/1(Lm_partial) -> M_partials/2(Lm_partial)
  M_partials/1(M0_partial) -> A_partial/3(M0_partial), M0_partial/1, AMA_partial/6(M0_partial), [M0_partial]
  A_partial/1(A_partial) -> AMA_partial/4(A_partial), [A_partial], A_partial1/1
  Constant/1 -> Lm_partials/2(Xi_m)
  M_partials/2(M0m_partial) -> A_partial/4(M0m_partial)
  Mm_hat_partial/1(Mm_hat_partial) -> C_hat1/2(Mm_hat_partial)
  q_dot_m1/1 -> C_hat1/3(q_dot_m)
  AMA_partial/1(AMA_partial) -> Mm_hat_partial/2(AMA_partial)
  <M0>/1 -> A_partial/2(M0)
  [V_I0] -> A_partial/6(V)
  [V_I0] -> M_partials/6(V)
  <Lm>/1 -> M_partials/4(Lm)
  [V_I0] -> AMA_partial/5(V)
  A/1 -> AMA_partial/3(A)
  C_hat1/1(C_hat) -> C_hat/1
  <M0>1/1 -> AMA_partial/2(M0)
  <Lm0>/1 -> M_partials/5(Lm0)

== system MMMS_v3/Feedback Transformation/Inverse Dynamics1/C_hat1 ==
  q_m : Inport
  q_dot_m : Inport  Port=2
  AMA_partial : MATLAB Function  TreatAsAtomicUnit=on
  A_partial : MATLAB Function  TreatAsAtomicUnit=on
  A_partial_par : MATLAB Function  TreatAsAtomicUnit=on
  Bus Selector : BusSelector  OutputSignals=M0,M0m
  Bus Selector1 : BusSelector  OutputSignals=Lm,Lm0
  C_hat : MATLAB Function  TreatAsAtomicUnit=on
  Constant : Constant  Value=Xi_m
  Constant2 : Constant  Commented=on  Value=m_diag  VectorParams1D=off
  Lm_partials : Subsystem
  M_partials : Subsystem
  Mm_hat_partial : MATLAB Function  TreatAsAtomicUnit=on
  M0_partial : Outport
  Out1 : Outport  Port=2
  C_hat1 : Outport  Port=3
  tag scope: A_partial=global, A_partial_par=global, M0_partial=global, Mm_partial=global
  wires:
  Bus Selector1/1 -> M_partials/4(Lm)  "<Lm>"
  M_partials/5(M0_partial_par) -> A_partial_par/7(M0_partial_par)
  M_partials/4(M0m_partial_par) -> A_partial_par/8(M0m_partial_par)
  M_partials/3(Mm_partial) -> [Mm_partial], Mm_hat_partial/3(Mm_partial)
  Lm_partials/4(Lm0_partial_par) -> M_partials/8(Lm0_partial_par)
  [L] -> Bus Selector1/1
  Bus Selector1/2 -> M_partials/5(Lm0)  "<Lm0>"
  AMA_partial/1(AMA_partial) -> Mm_hat_partial/2(AMA_partial)
  Lm_partials/2(Lm0_partial) -> M_partials/3(Lm0_partial)
  q_m/1 -> A_partial_par/1(q_m), AMA_partial/1(q_m), C_hat/1(q_m), Mm_hat_partial/1(q_m), A_partial/1(q_m), M_partials/1(q_m), Lm_partials/1(q_m)
  M_partials/1(M0_partial) -> AMA_partial/6(M0_partial), [M0_partial], M0_partial/1, A_partial/3(M0_partial), A_partial_par/3(M0_partial)
  Constant/1 -> Lm_partials/2(Xi_m)
  Mm_hat_partial/1(Mm_hat_partial) -> C_hat/2(Mm_hat_partial)
  Bus Selector/1 -> A_partial_par/2(M0), AMA_partial/2(M0), A_partial/2(M0)  "<M0>"
  [A_connection] -> AMA_partial/3(A)
  [V_Ie] -> AMA_partial/5(V)
  q_dot_m/1 -> C_hat/3(q_dot_m)
  [V_Ie] -> A_partial/6(V)
  [V_Ie] -> M_partials/7(V)
  Lm_partials/1(Lm_partial) -> M_partials/2(Lm_partial)
  Lm_partials/3(Lm_partial_par) -> M_partials/6(Lm_partial_par)
  [Mass_Matrix] -> Bus Selector/1
  [V_Ie] -> A_partial_par/6(V)
  Bus Selector/2 -> A_partial_par/5(M0m), A_partial/5(M0m)  "<M0m>"
  A_partial_par/1(A_partial_par) -> [A_partial_par]
  C_hat/1(C_hat) -> C_hat1/1
  M_partials/2(M0m_partial) -> A_partial_par/4(M0m_partial), A_partial/4(M0m_partial)
  A_partial/1(A_partial) -> Out1/1, [A_partial], AMA_partial/4(A_partial)

== system MMMS_v3/Feedback Transformation/Inverse Dynamics1/Inverse Dynamics ==
  note: Subsystem
  note: Inverse dynamics
  g_I0 : Inport
  <M0> : Inport  Port=2
  Mm : Inport  Port=3
  M0_dot : Inport  Port=4
  A_dot : Inport  Port=5
  C_hat : Inport  Port=6
  <M0>2 : InportShadow  Port=2
  Ad_g_I0_dot : MATLAB Function  TreatAsAtomicUnit=on
  Ad_g_I0_dot1 : MATLAB Function  TreatAsAtomicUnit=on
  Ad_g_te_dot : MATLAB Function  TreatAsAtomicUnit=on
  FU : MATLAB Function  TreatAsAtomicUnit=on
  Fm : MATLAB Function  TreatAsAtomicUnit=on
  Fmu : MATLAB Function  TreatAsAtomicUnit=on
  Gain : Gain  Commented=on  Gain=-1
  Goto : Goto  Commented=on  GotoTag=JJ  TagVisibility=global
  Inverse Dynamics : MATLAB Function  Commented=on  TreatAsAtomicUnit=on
  MATLAB Function3 : MATLAB Function  TreatAsAtomicUnit=on
  MmJcross : MATLAB Function  TreatAsAtomicUnit=on
  Mm_hat : MATLAB Function  TreatAsAtomicUnit=on
  Mt : Constant  Value=M_t
  Scope1 : Scope
  Scope2 : Scope
  F_U : Outport
  F_mu : Outport  Port=2
  F_t : Outport  Port=3
  F_m : Outport  Port=4
  tag scope: Mm_hat=global
  wires:
  Mm/1 -> Mm_hat/2(Mm)
  [A_connection] -> Mm_hat/3(A), MmJcross/2(A)
  FU/1(F_U) -> F_U/1
  Fmu/1(F_mu) -> F_mu/1
  MATLAB Function3/1(F_t) -> F_t/1
  Fm/1(F_m) -> F_m/1
  <M0>/1 -> Mm_hat/1(M0)
  C_hat/1 -> Fm/3(Cm_hat)
  <M0>2/1 -> Fmu/2(M0)
  g_I0/1 -> Fmu/4(g_I0), Ad_g_I0_dot/1(g_I0)
  M0_dot/1 -> Fmu/3(M_0_dot)
  A_dot/1 -> Fm/2(A_dot)
  [V_Ie] -> Ad_g_I0_dot/2(V_I0)
  Ad_g_I0_dot1/1(Ad_g_It_dot) -> MATLAB Function3/6(Ad_gIt_dot)
  Ad_g_I0_dot/1(Ad_g_I0_dot) -> Fmu/5(Ad_g_I0_dot)
  Ad_g_te_dot/1(Ad_g_te_dot) -> MATLAB Function3/5(Ad_gte_dot)
  [g_te] -> MATLAB Function3/2(g_te), Ad_g_te_dot/2(g_te)
  [g_It] -> MATLAB Function3/3(g_It), Ad_g_I0_dot1/2(g_It)
  [V_te] -> Ad_g_te_dot/1(V_te)
  [V_It] -> Ad_g_I0_dot1/1(V_t)
  Mt/1 -> MATLAB Function3/4(Mt)
  MmJcross/1(MmJcross) -> FU/1(MmJcross), MATLAB Function3/1(MmJcross), Fmu/1(MmJcross), Fm/1(MmJcross), Scope2/1
  Gain/1 -> Goto/1
  Mm_hat/1(Mm_hat) -> MmJcross/1(Mm_hat), [Mm_hat], Scope1/1

== system MMMS_v3/Feedback Transformation/Inverse Dynamics1/N_hat ==
  q_m : Inport
  q_dot_m : Inport  Port=2
  A : Inport  Port=3
  P : Inport  Port=4
  M0 : Inport  Port=5
  Constant : Constant  Value=iota0
  Matrix Multiply : Product  Multiplication=Matrix(*)
  N_hat : MATLAB Function  TreatAsAtomicUnit=on
  To Workspace : ToWorkspace  VariableName=N_firstpart  SaveFormat=Timeseries  SampleTime=-1
  N_hat1 : Outport
  wires:
  P/1 -> Matrix Multiply/2, N_hat/5(P)
  [M0_partial] -> N_hat/6(M0_partial)
  N_hat/1(N_hat_temp) -> To Workspace/1, Matrix Multiply/1
  q_m/1 -> N_hat/1(q_m)
  q_dot_m/1 -> N_hat/2(q_dot_m)
  [V_I0] -> N_hat/4(V)
  A/1 -> N_hat/3(A)
  [A_partial] -> N_hat/7(A_partial)
  Constant/1 -> N_hat/8(iota0)
  Matrix Multiply/1 -> N_hat1/1
  M0/1 -> N_hat/9(M0)

== system MMMS_v3/Feedback Transformation/Inverse Dynamics1/N_hat1 ==
  g_I0 : Inport
  q_m : Inport  Port=2
  q_dot_m : Inport  Port=3
  A : Inport  Port=4
  P : Inport  Port=5
  M0 : Inport  Port=6
  Constant : Constant  Value=iota0
  MATLAB Function : MATLAB Function  TreatAsAtomicUnit=on
  Matrix Multiply : Product  Multiplication=Matrix(*)
  N_hat : MATLAB Function  TreatAsAtomicUnit=on
  N_hat1 : Outport
  wires:
  [M0_partial] -> N_hat/6(M0_partial)
  N_hat/1(N_hat_temp) -> Matrix Multiply/1
  q_m/1 -> N_hat/1(q_m)
  q_dot_m/1 -> N_hat/2(q_dot_m)
  [V_Ie] -> MATLAB Function/2(V_Ie_e)
  A/1 -> N_hat/3(A)
  [A_partial] -> N_hat/7(A_partial)
  Constant/1 -> N_hat/8(iota0)
  Matrix Multiply/1 -> N_hat1/1
  M0/1 -> N_hat/9(M0)
  P/1 -> Matrix Multiply/2, N_hat/5(P)
  MATLAB Function/1(V_Ie) -> N_hat/4(V)
  g_I0/1 -> MATLAB Function/1(g_I0)

== system MMMS_v3/Feedback Transformation1/Inverse Dynamics1/C_hat ==
  note: C_hat
  q_m1 : Inport
  q_dot_m1 : Inport  Port=2
  A : Inport  Port=3
  <Lm0> : Inport  Port=4
  <Lm> : Inport  Port=5
  <M0> : Inport  Port=6
  <M0m> : Inport  Port=7
  <M0>1 : InportShadow  Port=6
  AMA_partial : MATLAB Function  TreatAsAtomicUnit=on
  A_partial : MATLAB Function  TreatAsAtomicUnit=on
  C_hat1 : MATLAB Function  TreatAsAtomicUnit=on
  Constant : Constant  Value=Xi_m
  Lm_partials : Subsystem
  M_partials : Subsystem
  Mm_hat_partial : MATLAB Function  TreatAsAtomicUnit=on
  M0_partial : Outport
  A_partial1 : Outport  Port=2
  C_hat : Outport  Port=3
  tag scope: A_partial=global, M0_partial=global
  wires:
  <Lm0>/1 -> M_partials/5(Lm0)
  <M0>1/1 -> AMA_partial/2(M0)
  C_hat1/1(C_hat) -> C_hat/1
  A/1 -> AMA_partial/3(A)
  [V_I0] -> AMA_partial/5(V)
  <Lm>/1 -> M_partials/4(Lm)
  [V_I0] -> M_partials/6(V)
  [V_I0] -> A_partial/6(V)
  <M0>/1 -> A_partial/2(M0)
  AMA_partial/1(AMA_partial) -> Mm_hat_partial/2(AMA_partial)
  q_dot_m1/1 -> C_hat1/3(q_dot_m)
  Mm_hat_partial/1(Mm_hat_partial) -> C_hat1/2(Mm_hat_partial)
  M_partials/2(M0m_partial) -> A_partial/4(M0m_partial)
  Constant/1 -> Lm_partials/2(Xi_m)
  A_partial/1(A_partial) -> A_partial1/1, [A_partial], AMA_partial/4(A_partial)
  M_partials/1(M0_partial) -> [M0_partial], AMA_partial/6(M0_partial), M0_partial/1, A_partial/3(M0_partial)
  Lm_partials/1(Lm_partial) -> M_partials/2(Lm_partial)
  <M0m>/1 -> A_partial/5(M0m)
  q_m1/1 -> M_partials/1(q_m), A_partial/1(q_m), AMA_partial/1(q_m), C_hat1/1(q_m), Mm_hat_partial/1(q_m), Lm_partials/1(q_m)
  Lm_partials/2(Lm0_partial) -> M_partials/3(Lm0_partial)
  M_partials/3(Mm_partial) -> Mm_hat_partial/3(Mm_partial)

== system MMMS_v3/Feedback Transformation1/Inverse Dynamics1/C_hat1 ==
  q_m1 : Inport
  q_dot_m1 : Inport  Port=2
  AMA_partial1 : MATLAB Function  TreatAsAtomicUnit=on
  A_partial1 : MATLAB Function  TreatAsAtomicUnit=on
  A_partial_par : MATLAB Function  TreatAsAtomicUnit=on
  Bus Selector2 : BusSelector  OutputSignals=M0,M0m
  Bus Selector3 : BusSelector  OutputSignals=Lm,Lm0
  C_hat2 : MATLAB Function  TreatAsAtomicUnit=on
  Constant1 : Constant  Value=Xi_m
  Constant3 : Constant  Commented=on  Value=m_diag  VectorParams1D=off
  Lm_partials1 : Subsystem
  M_partials1 : Subsystem
  Mm_hat_partial1 : MATLAB Function  TreatAsAtomicUnit=on
  M0_partial1 : Outport
  A_partial : Outport  Port=2
  C_hat3 : Outport  Port=3
  tag scope: A_partial2=global, A_partial_par2=global, M0_partial2=global, Mm_partial2=global
  wires:
  C_hat2/1(C_hat) -> C_hat3/1
  A_partial_par/1(A_partial_par) -> [A_partial_par2]
  [V_Ie2] -> AMA_partial1/5(V)
  Lm_partials1/1(Lm_partial) -> M_partials1/2(Lm_partial)
  [V_Ie2] -> A_partial_par/6(V)
  Mm_hat_partial1/1(Mm_hat_partial) -> C_hat2/2(Mm_hat_partial)
  M_partials1/2(M0m_partial) -> A_partial_par/4(M0m_partial), A_partial1/4(M0m_partial)
  Bus Selector2/1 -> A_partial_par/2(M0), AMA_partial1/2(M0), A_partial1/2(M0)  "<M0>"
  [Mass_Matrix2] -> Bus Selector2/1
  [A_connection2] -> AMA_partial1/3(A)
  Bus Selector2/2 -> A_partial_par/5(M0m), A_partial1/5(M0m)  "<M0m>"
  [V_Ie2] -> M_partials1/7(V)
  Constant1/1 -> Lm_partials1/2(Xi_m)
  Lm_partials1/2(Lm0_partial) -> M_partials1/3(Lm0_partial)
  M_partials1/1(M0_partial) -> AMA_partial1/6(M0_partial), [M0_partial2], M0_partial1/1, A_partial1/3(M0_partial), A_partial_par/3(M0_partial)
  Lm_partials1/3(Lm_partial_par) -> M_partials1/6(Lm_partial_par)
  q_m1/1 -> A_partial_par/1(q_m), AMA_partial1/1(q_m), C_hat2/1(q_m), Mm_hat_partial1/1(q_m), A_partial1/1(q_m), M_partials1/1(q_m), Lm_partials1/1(q_m)
  A_partial1/1(A_partial) -> [A_partial2], A_partial/1, AMA_partial1/4(A_partial)
  [L2] -> Bus Selector3/1
  [V_Ie2] -> A_partial1/6(V)
  q_dot_m1/1 -> C_hat2/3(q_dot_m)
  AMA_partial1/1(AMA_partial) -> Mm_hat_partial1/2(AMA_partial)
  M_partials1/3(Mm_partial) -> [Mm_partial2], Mm_hat_partial1/3(Mm_partial)
  M_partials1/5(M0_partial_par) -> A_partial_par/7(M0_partial_par)
  Bus Selector3/1 -> M_partials1/4(Lm)  "<Lm>"
  Bus Selector3/2 -> M_partials1/5(Lm0)  "<Lm0>"
  M_partials1/4(M0m_partial_par) -> A_partial_par/8(M0m_partial_par)
  Lm_partials1/4(Lm0_partial_par) -> M_partials1/8(Lm0_partial_par)

== system MMMS_v3/Feedback Transformation1/Inverse Dynamics1/Inverse Dynamics ==
  note: Inverse dynamics
  note: Subsystem
  g_I0 : Inport
  <M0> : Inport  Port=2
  Mm : Inport  Port=3
  M0_dot : Inport  Port=4
  A_dot : Inport  Port=5
  C_hat : Inport  Port=6
  <M0>2 : InportShadow  Port=2
  Ad_g_I0_dot : MATLAB Function  TreatAsAtomicUnit=on
  Ad_g_I0_dot1 : MATLAB Function  TreatAsAtomicUnit=on
  Ad_g_te_dot : MATLAB Function  TreatAsAtomicUnit=on
  FU : MATLAB Function  TreatAsAtomicUnit=on
  Fm : MATLAB Function  TreatAsAtomicUnit=on
  Fmu : MATLAB Function  TreatAsAtomicUnit=on
  MATLAB Function3 : MATLAB Function  TreatAsAtomicUnit=on
  MmJcross : MATLAB Function  TreatAsAtomicUnit=on
  Mm_hat : MATLAB Function  TreatAsAtomicUnit=on
  Mt : Constant  Value=M_t
  Scope1 : Scope
  Scope2 : Scope
  F_U : Outport
  F_mu : Outport  Port=2
  F_t : Outport  Port=3
  F_m : Outport  Port=4
  tag scope: Mm_hat2=global
  wires:
  MmJcross/1(MmJcross) -> Scope2/1, Fm/1(MmJcross), Fmu/1(MmJcross), MATLAB Function3/1(MmJcross), FU/1(MmJcross)
  Mt/1 -> MATLAB Function3/4(Mt)
  [V_It2] -> Ad_g_I0_dot1/1(V_t)
  [V_te2] -> Ad_g_te_dot/1(V_te)
  [g_It2] -> Ad_g_I0_dot1/2(g_It), MATLAB Function3/3(g_It)
  [g_te2] -> Ad_g_te_dot/2(g_te), MATLAB Function3/2(g_te)
  Ad_g_te_dot/1(Ad_g_te_dot) -> MATLAB Function3/5(Ad_gte_dot)
  Ad_g_I0_dot/1(Ad_g_I0_dot) -> Fmu/5(Ad_g_I0_dot)
  Ad_g_I0_dot1/1(Ad_g_It_dot) -> MATLAB Function3/6(Ad_gIt_dot)
  [V_Ie2] -> Ad_g_I0_dot/2(V_I0)
  A_dot/1 -> Fm/2(A_dot)
  M0_dot/1 -> Fmu/3(M_0_dot)
  g_I0/1 -> Ad_g_I0_dot/1(g_I0), Fmu/4(g_I0)
  <M0>2/1 -> Fmu/2(M0)
  C_hat/1 -> Fm/3(Cm_hat)
  <M0>/1 -> Mm_hat/1(M0)
  Fm/1(F_m) -> F_m/1
  MATLAB Function3/1(F_t) -> F_t/1
  Fmu/1(F_mu) -> F_mu/1
  FU/1(F_U) -> F_U/1
  [A_connection2] -> MmJcross/2(A), Mm_hat/3(A)
  Mm/1 -> Mm_hat/2(Mm)
  Mm_hat/1(Mm_hat) -> Scope1/1, [Mm_hat2], MmJcross/1(Mm_hat)

== system MMMS_v3/Feedback Transformation1/Inverse Dynamics1/N_hat ==
  q_m : Inport
  q_dot_m : Inport  Port=2
  A : Inport  Port=3
  P : Inport  Port=4
  M0 : Inport  Port=5
  Constant : Constant  Value=iota0
  Matrix Multiply : Product  Multiplication=Matrix(*)
  N_hat : MATLAB Function  TreatAsAtomicUnit=on
  To Workspace : ToWorkspace  VariableName=N_firstpart  SaveFormat=Timeseries  SampleTime=-1
  N_hat1 : Outport
  wires:
  M0/1 -> N_hat/9(M0)
  Matrix Multiply/1 -> N_hat1/1
  Constant/1 -> N_hat/8(iota0)
  [A_partial] -> N_hat/7(A_partial)
  A/1 -> N_hat/3(A)
  [V_I0] -> N_hat/4(V)
  q_dot_m/1 -> N_hat/2(q_dot_m)
  q_m/1 -> N_hat/1(q_m)
  N_hat/1(N_hat_temp) -> Matrix Multiply/1, To Workspace/1
  [M0_partial] -> N_hat/6(M0_partial)
  P/1 -> N_hat/5(P), Matrix Multiply/2

== system MMMS_v3/Feedback Transformation1/Inverse Dynamics1/N_hat1 ==
  g_I0 : Inport
  q_m : Inport  Port=2
  q_dot_m : Inport  Port=3
  A : Inport  Port=4
  P : Inport  Port=5
  M0 : Inport  Port=6
  Constant : Constant  Value=iota0
  MATLAB Function : MATLAB Function  TreatAsAtomicUnit=on
  Matrix Multiply : Product  Multiplication=Matrix(*)
  N_hat : MATLAB Function  TreatAsAtomicUnit=on
  N_hat1 : Outport
  wires:
  g_I0/1 -> MATLAB Function/1(g_I0)
  MATLAB Function/1(V_Ie) -> N_hat/4(V)
  P/1 -> N_hat/5(P), Matrix Multiply/2
  M0/1 -> N_hat/9(M0)
  Matrix Multiply/1 -> N_hat1/1
  Constant/1 -> N_hat/8(iota0)
  [A_partial2] -> N_hat/7(A_partial)
  A/1 -> N_hat/3(A)
  [V_Ie2] -> MATLAB Function/2(V_Ie_e)
  q_dot_m/1 -> N_hat/2(q_dot_m)
  q_m/1 -> N_hat/1(q_m)
  N_hat/1(N_hat_temp) -> Matrix Multiply/1
  [M0_partial2] -> N_hat/6(M0_partial)

== system MMMS_v3/Feedback Transformation2/Inverse Dynamics1/C_hat ==
  note: C_hat
  q_m1 : Inport
  q_dot_m1 : Inport  Port=2
  A : Inport  Port=3
  <Lm0> : Inport  Port=4
  <Lm> : Inport  Port=5
  <M0> : Inport  Port=6
  <M0m> : Inport  Port=7
  <M0>1 : InportShadow  Port=6
  AMA_partial : MATLAB Function  TreatAsAtomicUnit=on
  A_partial : MATLAB Function  TreatAsAtomicUnit=on
  C_hat1 : MATLAB Function  TreatAsAtomicUnit=on
  Constant : Constant  Value=Xi_m
  Lm_partials : Subsystem
  M_partials : Subsystem
  Mm_hat_partial : MATLAB Function  TreatAsAtomicUnit=on
  M0_partial : Outport
  A_partial1 : Outport  Port=2
  C_hat : Outport  Port=3
  tag scope: A_partial=global, M0_partial=global
  wires:
  M_partials/3(Mm_partial) -> Mm_hat_partial/3(Mm_partial)
  Lm_partials/2(Lm0_partial) -> M_partials/3(Lm0_partial)
  q_m1/1 -> Lm_partials/1(q_m), Mm_hat_partial/1(q_m), C_hat1/1(q_m), AMA_partial/1(q_m), A_partial/1(q_m), M_partials/1(q_m)
  <M0m>/1 -> A_partial/5(M0m)
  Lm_partials/1(Lm_partial) -> M_partials/2(Lm_partial)
  M_partials/1(M0_partial) -> A_partial/3(M0_partial), M0_partial/1, AMA_partial/6(M0_partial), [M0_partial]
  A_partial/1(A_partial) -> AMA_partial/4(A_partial), [A_partial], A_partial1/1
  Constant/1 -> Lm_partials/2(Xi_m)
  M_partials/2(M0m_partial) -> A_partial/4(M0m_partial)
  Mm_hat_partial/1(Mm_hat_partial) -> C_hat1/2(Mm_hat_partial)
  q_dot_m1/1 -> C_hat1/3(q_dot_m)
  AMA_partial/1(AMA_partial) -> Mm_hat_partial/2(AMA_partial)
  <M0>/1 -> A_partial/2(M0)
  [V_I0] -> A_partial/6(V)
  [V_I0] -> M_partials/6(V)
  <Lm>/1 -> M_partials/4(Lm)
  [V_I0] -> AMA_partial/5(V)
  A/1 -> AMA_partial/3(A)
  C_hat1/1(C_hat) -> C_hat/1
  <M0>1/1 -> AMA_partial/2(M0)
  <Lm0>/1 -> M_partials/5(Lm0)
